simulink model "question8_2015a"  (R2015a)
settings: Solver=ode45  SolverMode=SingleTasking  StartTime=0.0  StopTime=T  RelTol=1e-3
values from neighbouring files (symbols this model uses):
  A_c = A - B*K - L*C    [hw.m]
  B_c = L    [hw.m]
  C_c = -K    [hw.m]
  D = [0 0]'    [hw.m]
  D_c = zeros(size(C_c,1), size(B_c,2))    [hw.m]
  x0 = [1 0 1 0 0]'    [hw.m]
undefined symbols (not defined in the file or in its folder): A, B, C
settings Model: CovMetricSettings=dwe  CovHtmlReporting=off  covSaveCumulativeToWorkspaceVar=off  CovSaveSingleToWorkspaceVar=off  CovExternalEMLEnable=on  Creator=antonio  LastModifiedBy=antonio
settings DataIOCC: LimitDataPoints=off  SaveFormat=Dataset  ReturnWorkspaceOutputs=on
settings DebuggingCC: UnconnectedInputMsg=none  UnconnectedOutputMsg=none  UnconnectedLineMsg=none  SFUnexpectedBacktrackingDiag=error  SFNoUnconditionalDefaultTransitionDiag=error
settings HardwareCC: ProdBitPerPointer=64  ProdLargestAtomicFloat=Float  ProdIntDivRoundTo=Zero  ProdEndianess=LittleEndian  ProdHWDeviceType=Specified
settings ModelReferenceCC: PropagateSignalLabelsOutOfModel=on
settings SFSimCC: SimUseLocalCustomCode=on
settings RTWCC: RTWUseLocalCustomCode=on
settings GRTTargetCC: TargetLangStandard=C99 (ISO)

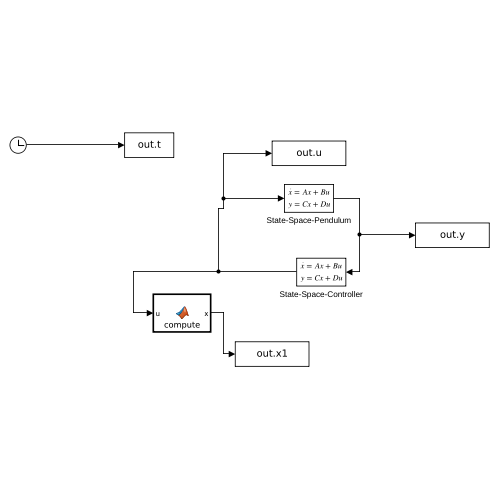
[thumbnail: Simulink's stored preview of the top-level diagram]
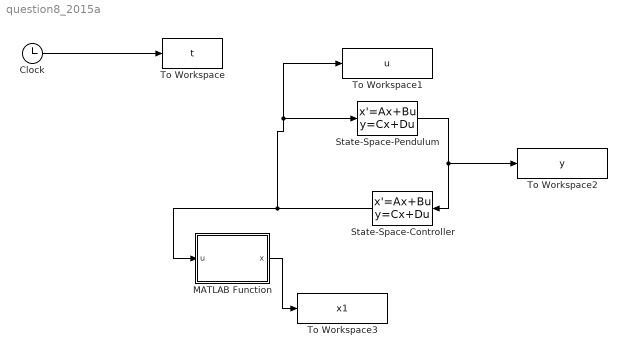
== system question8_2015a ==
  Clock : Clock
  MATLAB Function : MATLAB Function  TreatAsAtomicUnit=on
      settings: PermitHierarchicalResolution=ParametersOnly
  State-Space-Controller : StateSpace  A=A_c  B=B_c  C=C_c  D=D_c  X0=x0  ContinuousStateAttributes='State'
  State-Space-Pendulum : StateSpace  A=A  B=B  C=C  D=D  X0=x0  ContinuousStateAttributes='State'
  To Workspace : ToWorkspace  VariableName=t  SampleTime=-1
  To Workspace1 : ToWorkspace  VariableName=u  SampleTime=-1
  To Workspace2 : ToWorkspace  VariableName=y  SampleTime=-1
  To Workspace3 : ToWorkspace  VariableName=x1  SampleTime=-1
  wires:
  Clock/1 -> To Workspace/1
  State-Space-Pendulum/1 -> State-Space-Controller/1, To Workspace2/1
  State-Space-Controller/1 -> MATLAB Function/1(u), To Workspace1/1, State-Space-Pendulum/1
  MATLAB Function/1(x) -> To Workspace3/1

== matlab function question8_2015a/MATLAB Function ==
  data: u input; x output
function x = compute(u)
    K = [-3.1623,-3.0458,30.3790,4.5686,0.3142];
    K_pinv = pinv(K);
    x = -K_pinv * u;

end
